simulink model "NonLinear_MotorControl"  (R2017b)
settings: Solver=ode4  StartTime=0.0  StopTime=10  FixedStep=0.0001  MaxStep=0.001  MinStep=0.0001  RelTol=1e-3
(part 1 of 2)
settings Model: Creator=ASUS  LastModifiedBy=ASUS
settings SolverCC: ShapePreserveControl=EnableAll  ZeroCrossAlgorithm=Adaptive

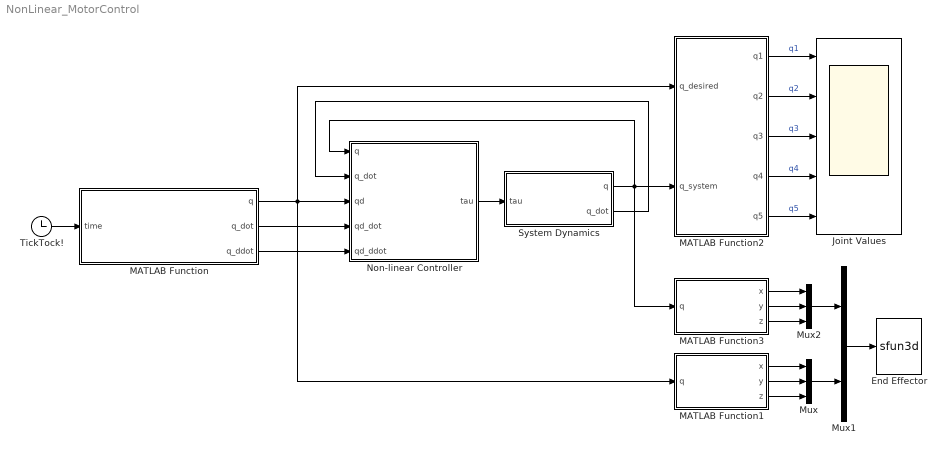
== system NonLinear_MotorControl ==
  End Effector : S-Function  LoadFcn=if exist('sfun3d','file'), sfun3d([],[],[],'LoadBlock'); end  FunctionName=sfun3d  Parameters=ax,T,np,cp,gd,ls,mk,mx,hd,tb  SFunctionDeploymentMode=off  EnableBusSupport=off  mask(3D Graph){np=2, ax=[-450 450 -2000 0 -4000 -500], mx=1e4, T=0.001, cp=[-450 -2000 -500], gd=on, hd=on, tb=on, ls=-, mk=none}
      mask prompts: np "Number of moving points (lines)"; ax "Range: [xmin xmax  ymin ymax zmin zmax]"; mx "Max number of points in each line"; T "Sampling Time"; cp "Camera position (use [0 0 1] for 2D XY view)"; gd "Grid (on|off)"; hd "HeadMarkers (on|off)"; tb "Toolbar (on|off)"; ls "LineStyle"; mk "LineMarker"
      mask help:
      | This block plots the position of several points in the XYZ space. The input contains the coordinates of all the points (x1,y1,z1,x2,y2,z2,...).
      | The number of moving points (lines), the XYZ ranges, sampling time, camera position, and grid (among other things) can be set as mask parameters.
      settings: CopyFcn=if exist('sfun3d','file'), sfun3d([],[],[],'CopyBlock'); end  DeleteFcn=if exist('sfun3d','file'), sfun3d([],[],[],'DeleteBlock'); end  NameChangeFcn=if exist('sfun3d','file'), sfun3d([],[],[],'NameChange'); end
      mask Help:
      | This block plots the position of several points in the XYZ space. The input contains the coordinates of all the points (x1,y1,z1,x2,y2,z2,...).
      | The number of moving points (lines), the XYZ ranges, sampling time, camera position, and grid (among other things) can be set as mask parameters.
      mask TypeOptions ls: - | -- | : | -. | none
      mask TypeOptions mk: none | . | + | o | * | x | square | diamond | v | ^ | > | < | pentagram | hexagram
      mask Display: plot([.05 .95 .95 .05 .05],[.45 .45 .95 .95 .45], 0.5+cos(0:0.1:2*pi)*0.3,0.7+sin(0:0.1:2*pi)*0.2)
  Joint Values : Scope  NumInputPorts=5
  MATLAB Function : MATLAB Function  TreatAsAtomicUnit=on
  MATLAB Function1 : MATLAB Function  TreatAsAtomicUnit=on
  MATLAB Function2 : MATLAB Function  TreatAsAtomicUnit=on
  MATLAB Function3 : MATLAB Function  TreatAsAtomicUnit=on
  Mux : Mux  Inputs=3
  Mux1 : Mux  Inputs=2
  Mux2 : Mux  Inputs=3
  Non-linear Controller : MATLAB Function  TreatAsAtomicUnit=on
  System Dynamics : Subsystem
  TickTock! : Clock
  wires:
  Non-linear Controller/1(tau) -> System Dynamics/1(tau)
  System Dynamics/2(q_dot) -> Non-linear Controller/2(q_dot)
  TickTock!/1 -> MATLAB Function/1(time)
  MATLAB Function/2(q_dot) -> Non-linear Controller/4(qd_dot)
  MATLAB Function/3(q_ddot) -> Non-linear Controller/5(qd_ddot)
  System Dynamics/1(q) -> Non-linear Controller/1(q), MATLAB Function2/2(q_system), MATLAB Function3/1(q)
  MATLAB Function/1(q) -> Non-linear Controller/3(qd), MATLAB Function2/1(q_desired), MATLAB Function1/1(q)
  MATLAB Function1/2(y) -> Mux/2
  MATLAB Function1/1(x) -> Mux/1
  MATLAB Function1/3(z) -> Mux/3
  Mux/1 -> Mux1/2
  Mux1/1 -> End Effector/1
  MATLAB Function3/1(x) -> Mux2/1
  MATLAB Function3/2(y) -> Mux2/2
  MATLAB Function3/3(z) -> Mux2/3
  Mux2/1 -> Mux1/1
  MATLAB Function2/1(q1) -> Joint Values/1  "q1"
  MATLAB Function2/2(q2) -> Joint Values/2  "q2"
  MATLAB Function2/3(q3) -> Joint Values/3  "q3"
  MATLAB Function2/4(q4) -> Joint Values/4  "q4"
  MATLAB Function2/5(q5) -> Joint Values/5  "q5"

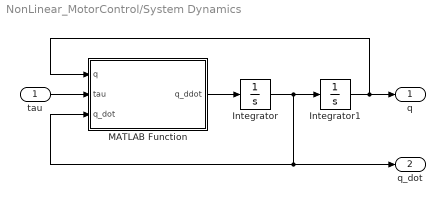
== system NonLinear_MotorControl/System Dynamics ==
  tau : Inport
  Integrator : Integrator  InitialCondition=zeros(5,1)
  Integrator1 : Integrator  InitialCondition=[1 -pi/18 10 0 0]'
  MATLAB Function : MATLAB Function  TreatAsAtomicUnit=on
  q : Outport
  q_dot : Outport  Port=2
  wires:
  MATLAB Function/1(q_ddot) -> Integrator/1
  Integrator1/1 -> q/1, MATLAB Function/1(q)
  Integrator/1 -> Integrator1/1, q_dot/1, MATLAB Function/3(q_dot)
  tau/1 -> MATLAB Function/2(tau)

== matlab function NonLinear_MotorControl/Non-linear Controller ==
  data: q input; tau output; q_dot input; qd input; qd_dot input; qd_ddot input
function tau = ctrl(q,q_dot,qd,qd_dot,qd_ddot)
   q_1 = q(1);
   q_2 = q(2);
   q_3 = q(3);
   q_4 = q(4);
   q_5 = q(5);
    
   %% M
   M = ...
[                                                                                                                                                                                                                                                                                                                                                                                                                                                                                                                                                                                                                                                                                                                                                                                                               243/2,                                                                                                                                                                                                                               (1637253847765431*cos(q_2 + q_4 + q_5))/2748779069440 + (3015813*sin(q_2 + q_4 + q_5))/12500 + (1637253847765431*cos(q_2 + q_4 - q_5))/2748779069440 + (3015813*sin(q_2 + q_4 - q_5))/12500 - (1637253847765431*cos(q_2 + q_4))/1374389534720 + (13930449*cos(q_2))/500000 + (11396226878722115871*sin(q_2))/1759218604441600 - (1637253847765431*2^(1/2)*cos(q_2 + q_4 - q_5))/2748779069440 - (3015813*2^(1/2)*sin(q_2 + q_4 - q_5))/25000 - (3567380807909369503983*2^(1/2)*cos(q_2 + q_4))/2199023255552000000 + (1637253847765431*2^(1/2)*cos(q_2 + q_4 + q_5))/2748779069440 + (3015813*2^(1/2)*sin(q_2 + q_4 + q_5))/25000,                                                                            0,                                                                                                                                                                                                                                                                                                               (1637253847765431*cos(q_2 + q_4 + q_5))/2748779069440 + (3015813*sin(q_2 + q_4 + q_5))/12500 + (1637253847765431*cos(q_2 + q_4 - q_5))/2748779069440 + (3015813*sin(q_2 + q_4 - q_5))/12500 - (1637253847765431*cos(q_2 + q_4))/1374389534720 - (1637253847765431*2^(1/2)*cos(q_2 + q_4 - q_5))/2748779069440 - (3015813*2^(1/2)*sin(q_2 + q_4 - q_5))/25000 - (3567380807909369503983*2^(1/2)*cos(q_2 + q_4))/2199023255552000000 + (1637253847765431*2^(1/2)*cos(q_2 + q_4 + q_5))/2748779069440 + (3015813*2^(1/2)*sin(q_2 + q_4 + q_5))/25000,                                                                                           (1637253847765431*cos(q_2 + q_4 + q_5))/2748779069440 + (3015813*sin(q_2 + q_4 + q_5))/12500 - (1637253847765431*cos(q_2 + q_4 - q_5))/2748779069440 - (3015813*sin(q_2 + q_4 - q_5))/12500 + (1637253847765431*2^(1/2)*cos(q_2 + q_4 - q_5))/2748779069440 + (3015813*2^(1/2)*sin(q_2 + q_4 - q_5))/25000 + (1637253847765431*2^(1/2)*cos(q_2 + q_4 + q_5))/2748779069440 + (3015813*2^(1/2)*sin(q_2 + q_4 + q_5))/25000
  (13930449*cos(q_2))/500000 + (11396226878722115871*sin(q_2))/1759218604441600 - (1637253847765431*cos(q_2)*cos(q_4))/1374389534720 + (1637253847765431*sin(q_2)*sin(q_4))/1374389534720 - (3567380807909369503983*2^(1/2)*cos(q_2)*cos(q_4))/2199023255552000000 + (3567380807909369503983*2^(1/2)*sin(q_2)*sin(q_4))/2199023255552000000 + (1637253847765431*cos(q_2)*cos(q_4)*cos(q_5))/1374389534720 + (3015813*cos(q_2)*cos(q_5)*sin(q_4))/6250 + (3015813*cos(q_4)*cos(q_5)*sin(q_2))/6250 - (1637253847765431*cos(q_5)*sin(q_2)*sin(q_4))/1374389534720 + (3015813*2^(1/2)*cos(q_2)*cos(q_4)*sin(q_5))/12500 - (1637253847765431*2^(1/2)*cos(q_2)*sin(q_4)*sin(q_5))/1374389534720 - (1637253847765431*2^(1/2)*cos(q_4)*sin(q_2)*sin(q_5))/1374389534720 - (3015813*2^(1/2)*sin(q_2)*sin(q_4)*sin(q_5))/12500,  sin(q_5)/1000 - (47028073017942265058105238873*cos(q_5))/151115727451828646838272 - (1637253847765431*sin(q_4))/1374389534720 - (57*sin(2*q_5))/2000 - (86625503688717695659*2^(1/2)*sin(2*q_5))/2748779069440000 - (3015813*cos(q_4)*cos(q_5))/6250 + (1637253847765431*cos(q_5)*sin(q_4))/1374389534720 - (25261205975153249495668933896699961*cos(q_5)^2)/118059162071741130342400000000 + (21357421969732009*2^(1/2))/549755813888 + (3796988859053507*2^(1/2)*cos(q_5))/549755813888 - (3567380807909369503983*2^(1/2)*sin(q_4))/2199023255552000000 - (86625502314328160939*2^(1/2)*sin(q_5))/1374389534720000 - (16938612281049*2^(1/2)*cos(q_5)^2)/68719476736 + (1637253847765431*2^(1/2)*cos(q_4)*sin(q_5))/1374389534720 + (3015813*2^(1/2)*sin(q_4)*sin(q_5))/12500 + 31233135728824415250615508218939171019991/4835703278458516698824704000000000,                                                                            0, sin(q_5)/1000 - (47028073017942265058105238873*cos(q_5))/151115727451828646838272 - (1637253847765431*sin(q_4))/2748779069440 - (57*sin(2*q_5))/2000 - (86625503688717695659*2^(1/2)*sin(2*q_5))/2748779069440000 - (3015813*cos(q_4)*cos(q_5))/12500 + (1637253847765431*cos(q_5)*sin(q_4))/2748779069440 - (25261205975153249495668933896699961*cos(q_5)^2)/118059162071741130342400000000 + (21357421969732009*2^(1/2))/549755813888 + (3796988859053507*2^(1/2)*cos(q_5))/549755813888 - (3567380807909369503983*2^(1/2)*sin(q_4))/4398046511104000000 - (86625502314328160939*2^(1/2)*sin(q_5))/1374389534720000 - (16938612281049*2^(1/2)*cos(q_5)^2)/68719476736 + (1637253847765431*2^(1/2)*cos(q_4)*sin(q_5))/2748779069440 + (3015813*2^(1/2)*sin(q_4)*sin(q_5))/25000 + 10245887604910058238243681116147296112739/4835703278458516698824704000000000, (1637253847765431*cos(q_4)*sin(q_5))/2748779069440 - (86625463831421188779*sin(q_5))/1374389534720000 - (8712462106215055*cos(q_5))/274877906944 + (3015813*sin(q_4)*sin(q_5))/12500 + (19877377088082943877744654372831289*2^(1/2))/118059162071741130342400000000 - (47028073017942265058105238873*2^(1/2)*cos(q_5))/302231454903657293676544 + (2^(1/2)*sin(q_5))/1000 - (3015813*2^(1/2)*cos(q_4)*cos(q_5))/25000 + (1637253847765431*2^(1/2)*cos(q_5)*sin(q_4))/2748779069440 + 21357421969732009/274877906944
                                                                                                                                                                                                                                                                                                                                                                                                                                                                                                                                                                                                                                                                                                                                                                                                                    0,                                                                                                                                                                                                                                                                                                                                                                                                                                                                                                                                                                                                                                                                                                                                                                                                                                                               0,                                                                      1539/40,                                                                                                                                                                                                                                                                                                                                                                                                                                                                                                                                                                                                                                                                                                                                                                                                                                                               0,                                                                                                                                                                                                                                                                                                                                                                                                                                        (1637253847765431*sin(q_5))/1374389534720 - (3015813*2^(1/2)*cos(q_5))/12500
                                                                                  (1637253847765431*sin(q_2)*sin(q_4))/1374389534720 - (1637253847765431*cos(q_2)*cos(q_4))/1374389534720 - (3567380807909369503983*2^(1/2)*cos(q_2)*cos(q_4))/2199023255552000000 + (3567380807909369503983*2^(1/2)*sin(q_2)*sin(q_4))/2199023255552000000 + (1637253847765431*cos(q_2)*cos(q_4)*cos(q_5))/1374389534720 + (3015813*cos(q_2)*cos(q_5)*sin(q_4))/6250 + (3015813*cos(q_4)*cos(q_5)*sin(q_2))/6250 - (1637253847765431*cos(q_5)*sin(q_2)*sin(q_4))/1374389534720 + (3015813*2^(1/2)*cos(q_2)*cos(q_4)*sin(q_5))/12500 - (1637253847765431*2^(1/2)*cos(q_2)*sin(q_4)*sin(q_5))/1374389534720 - (1637253847765431*2^(1/2)*cos(q_4)*sin(q_2)*sin(q_5))/1374389534720 - (3015813*2^(1/2)*sin(q_2)*sin(q_4)*sin(q_5))/12500, sin(q_5)/1000 - (47028073017942265058105238873*cos(q_5))/151115727451828646838272 - (1637253847765431*sin(q_4))/2748779069440 - (57*sin(2*q_5))/2000 - (86625503688717695659*2^(1/2)*sin(2*q_5))/2748779069440000 - (3015813*cos(q_4)*cos(q_5))/12500 + (1637253847765431*cos(q_5)*sin(q_4))/2748779069440 - (25261205975153249495668933896699961*cos(q_5)^2)/118059162071741130342400000000 + (21357421969732009*2^(1/2))/549755813888 + (3796988859053507*2^(1/2)*cos(q_5))/549755813888 - (3567380807909369503983*2^(1/2)*sin(q_4))/4398046511104000000 - (86625502314328160939*2^(1/2)*sin(q_5))/1374389534720000 - (16938612281049*2^(1/2)*cos(q_5)^2)/68719476736 + (1637253847765431*2^(1/2)*cos(q_4)*sin(q_5))/2748779069440 + (3015813*2^(1/2)*sin(q_4)*sin(q_5))/25000 + 10245887604910058238243681116147296112739/4835703278458516698824704000000000,                                                                            0,                                                                                                                                                                                                                                                                                                               sin(q_5)/1000 - (47028073017942265058105238873*cos(q_5))/151115727451828646838272 - (57*sin(2*q_5))/2000 - (86625503688717695659*2^(1/2)*sin(2*q_5))/2748779069440000 - (25261205975153249495668933896699961*cos(q_5)^2)/118059162071741130342400000000 + (21357421969732009*2^(1/2))/549755813888 + (3796988859053507*2^(1/2)*cos(q_5))/549755813888 - (86625502314328160939*2^(1/2)*sin(q_5))/1374389534720000 - (16938612281049*2^(1/2)*cos(q_5)^2)/68719476736 + 10245887604910058238243681116147296112739/4835703278458516698824704000000000,                                                                                                                                                                                                   (19877377088082943877744654372831289*2^(1/2))/118059162071741130342400000000 - (86625463831421188779*sin(q_5))/1374389534720000 - (8712462106215055*cos(q_5))/274877906944 - (47028073017942265058105238873*2^(1/2)*cos(q_5))/302231454903657293676544 + (2^(1/2)*sin(q_5))/1000 + 21357421969732009/274877906944
                                                                                                                                                                                                                                                                                                                                              (3015813*cos(q_2)*cos(q_4)*sin(q_5))/6250 - (3015813*sin(q_2)*sin(q_4)*sin(q_5))/6250 - (1637253847765431*cos(q_2)*sin(q_4)*sin(q_5))/1374389534720 - (1637253847765431*cos(q_4)*sin(q_2)*sin(q_5))/1374389534720 + (1637253847765431*2^(1/2)*cos(q_2)*cos(q_4)*cos(q_5))/1374389534720 + (3015813*2^(1/2)*cos(q_2)*cos(q_5)*sin(q_4))/12500 + (3015813*2^(1/2)*cos(q_4)*cos(q_5)*sin(q_2))/12500 - (1637253847765431*2^(1/2)*cos(q_5)*sin(q_2)*sin(q_4))/1374389534720,                                                                                                                                                                                                                                                                                                                                                                       (6254725482634281*cos(q_5))/137438953472 - (86625540797235133099*sin(q_5))/1374389534720000 + (1637253847765431*cos(q_4)*sin(q_5))/2748779069440 + (3015813*sin(q_4)*sin(q_5))/12500 + (19877377088082943877744654372831289*2^(1/2))/118059162071741130342400000000 - (47028073017942265058105238873*2^(1/2)*cos(q_5))/302231454903657293676544 - (3015813*2^(1/2)*cos(q_4)*cos(q_5))/25000 + (1637253847765431*2^(1/2)*cos(q_5)*sin(q_4))/2748779069440 + 21357421969732009/274877906944, (1637253847765431*sin(q_5))/1374389534720 - (3015813*2^(1/2)*cos(q_5))/12500,                                                                                                                                                                                                                                                                                                                                                                                                                                                                                                                                                                         (6254725482634281*cos(q_5))/137438953472 - (86625540797235133099*sin(q_5))/1374389534720000 + (19877377088082943877744654372831289*2^(1/2))/118059162071741130342400000000 - (47028073017942265058105238873*2^(1/2)*cos(q_5))/302231454903657293676544 + 21357421969732009/274877906944,                                                                                                                                                                                                                                                                                                                                                                                                        (21357421969732009*2^(1/2))/274877906944 + 19877377088082943877744654372831289/59029581035870565171200000000];
 
   %% C
   C = ...
[ 0,                                            (3015813*cos(q_2 + q_4 + q_5))/12500 - (1637253847765431*sin(q_2 + q_4 + q_5))/2748779069440 + (3015813*cos(q_2 + q_4 - q_5))/12500 - (1637253847765431*sin(q_2 + q_4 - q_5))/2748779069440 + (1637253847765431*sin(q_2 + q_4))/1374389534720 + (11396226878722115871*cos(q_2))/1759218604441600 - (13930449*sin(q_2))/500000 - (3015813*2^(1/2)*cos(q_2 + q_4 - q_5))/25000 + (1637253847765431*2^(1/2)*sin(q_2 + q_4 - q_5))/2748779069440 + (3567380807909369503983*2^(1/2)*sin(q_2 + q_4))/2199023255552000000 + (3015813*2^(1/2)*cos(q_2 + q_4 + q_5))/25000 - (1637253847765431*2^(1/2)*sin(q_2 + q_4 + q_5))/2748779069440, 0, (3015813*cos(q_2 + q_4 + q_5))/12500 - (1637253847765431*sin(q_2 + q_4 + q_5))/2748779069440 + (3015813*cos(q_2 + q_4 - q_5))/12500 - (1637253847765431*sin(q_2 + q_4 - q_5))/2748779069440 + (1637253847765431*sin(q_2 + q_4))/1374389534720 - (3015813*2^(1/2)*cos(q_2 + q_4 - q_5))/25000 + (1637253847765431*2^(1/2)*sin(q_2 + q_4 - q_5))/2748779069440 + (3567380807909369503983*2^(1/2)*sin(q_2 + q_4))/2199023255552000000 + (3015813*2^(1/2)*cos(q_2 + q_4 + q_5))/25000 - (1637253847765431*2^(1/2)*sin(q_2 + q_4 + q_5))/2748779069440, (3015813*cos(q_2 + q_4 + q_5))/12500 - (1637253847765431*sin(q_2 + q_4 + q_5))/2748779069440 + (3015813*cos(q_2 + q_4 - q_5))/12500 - (1637253847765431*sin(q_2 + q_4 - q_5))/2748779069440 - (3015813*2^(1/2)*cos(q_2 + q_4 - q_5))/25000 + (1637253847765431*2^(1/2)*sin(q_2 + q_4 - q_5))/2748779069440 + (3015813*2^(1/2)*cos(q_2 + q_4 + q_5))/25000 - (1637253847765431*2^(1/2)*sin(q_2 + q_4 + q_5))/2748779069440
  0,                                                                                                                                                                                                                                                                                                                                                                                                                                                                                                                                                                                                                                                                            0, 0,                                                                                                                                                                                                                                       (1637253847765431*cos(q_4)*cos(q_5))/2748779069440 - (1637253847765431*cos(q_4))/2748779069440 + (3015813*cos(q_5)*sin(q_4))/12500 - (3567380807909369503983*2^(1/2)*cos(q_4))/4398046511104000000 + (3015813*2^(1/2)*cos(q_4)*sin(q_5))/25000 - (1637253847765431*2^(1/2)*sin(q_4)*sin(q_5))/2748779069440,                       (8712462106215055*sin(q_5))/274877906944 - (86625463831421188779*cos(q_5))/1374389534720000 + (1637253847765431*cos(q_4)*cos(q_5))/2748779069440 + (3015813*cos(q_5)*sin(q_4))/12500 + (2^(1/2)*cos(q_5))/1000 + (47028073017942265058105238873*2^(1/2)*sin(q_5))/302231454903657293676544 + (3015813*2^(1/2)*cos(q_4)*sin(q_5))/25000 - (1637253847765431*2^(1/2)*sin(q_4)*sin(q_5))/2748779069440
  0,                                                                                                                                                                                                                                                                                                                                                                                                                                                                                                                                                                                                                                                                            0, 0,                                                                                                                                                                                                                                                                                                                                                                                                                                                                                                                                                 0,                                                                                                                                                                                                                                                                                                                                              (1637253847765431*cos(q_5))/1374389534720 + (3015813*2^(1/2)*sin(q_5))/12500
  0,                                                                                                                                                                                                                                                                                                                                                                  (1637253847765431*cos(q_4))/2748779069440 - (1637253847765431*cos(q_4)*cos(q_5))/2748779069440 - (3015813*cos(q_5)*sin(q_4))/12500 + (3567380807909369503983*2^(1/2)*cos(q_4))/4398046511104000000 - (3015813*2^(1/2)*cos(q_4)*sin(q_5))/25000 + (1637253847765431*2^(1/2)*sin(q_4)*sin(q_5))/2748779069440, 0,                                                                                                                                                                                                                                                                                                                                                                                                                                                                                                                                                 0,                                                                                                                                                                                                                         (8712462106215055*sin(q_5))/274877906944 - (86625463831421188779*cos(q_5))/1374389534720000 + (2^(1/2)*cos(q_5))/1000 + (47028073017942265058105238873*2^(1/2)*sin(q_5))/302231454903657293676544
  0, (1637253847765431*sin(q_4)*sin(q_5))/2748779069440 - cos(q_5)/1000 - (47028073017942265058105238873*sin(q_5))/302231454903657293676544 - (16938612281049*2^(1/2)*sin(2*q_5))/137438953472 - (3015813*cos(q_4)*sin(q_5))/12500 - (25261205975153249495668933896699961*sin(2*q_5))/236118324143482260684800000000 + (57*cos(q_5)^2)/1000 - (86625543546014202539*2^(1/2))/2748779069440000 + (86625463831421188779*2^(1/2)*cos(q_5))/2748779069440000 - (8712462106215055*2^(1/2)*sin(q_5))/549755813888 + (86625503688717695659*2^(1/2)*cos(q_5)^2)/1374389534720000 - (1637253847765431*2^(1/2)*cos(q_4)*cos(q_5))/2748779069440 - (3015813*2^(1/2)*cos(q_5)*sin(q_4))/25000, 0,                                                                        (57*cos(q_5)^2)/1000 - cos(q_5)/1000 - (47028073017942265058105238873*sin(q_5))/302231454903657293676544 - (16938612281049*2^(1/2)*sin(2*q_5))/137438953472 - (25261205975153249495668933896699961*sin(2*q_5))/236118324143482260684800000000 - (86625543546014202539*2^(1/2))/2748779069440000 + (86625463831421188779*2^(1/2)*cos(q_5))/2748779069440000 - (8712462106215055*2^(1/2)*sin(q_5))/549755813888 + (86625503688717695659*2^(1/2)*cos(q_5)^2)/1374389534720000,                                                                                                                                                                                                                                                                                                                                                                                                                         0];
 
   %% G
   G = ...
[ 
                                                                                      0
                                                                                      0
                                                                          -1509759/4000
                                                                                      0
 (2958512553*2^(1/2)*cos(q_5))/1250000 - (1606146024657887811*sin(q_5))/137438953472000];

   %% Controller
   a   = qd_ddot + 10*(qd_dot - q_dot) + 25*(qd - q);
   tau = M*a + C*q_dot + G;
end
